simulink model "gridfor575V"  (R2015b)
settings: Solver=VariableStepAuto  StartTime=0.0  StopTime=10.0  RelTol=1e-3
values from neighbouring files (symbols this model uses):
  Ts = 5E-6    (= 5e-06)    [GE275103_inertial_support.m]
libraries: powerlib x8, sps_avr x1, powerlib_meascontrol x1
settings Model: Creator=Eren  LastModifiedBy=Eren

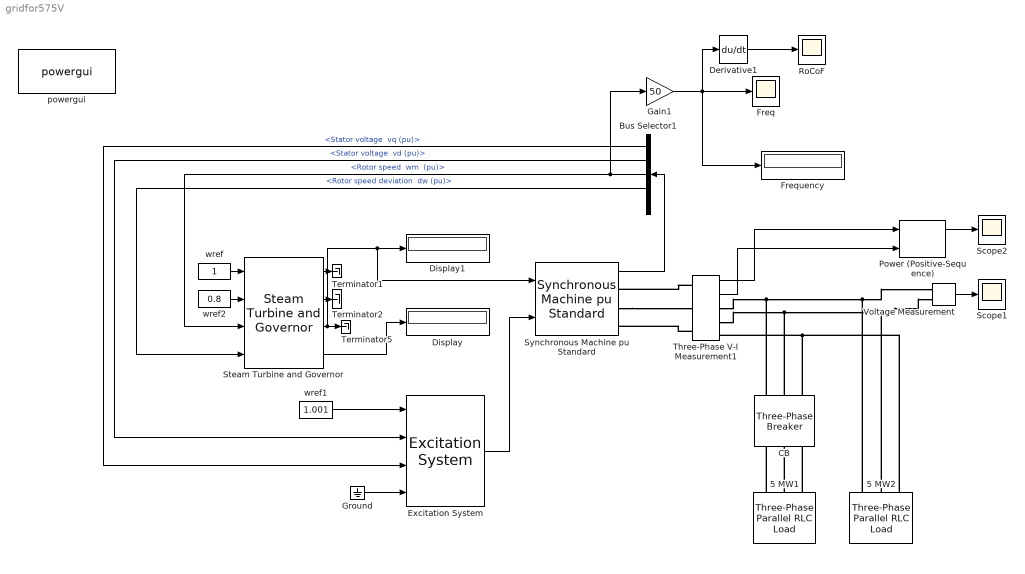
== system gridfor575V ==
  5 MW1 : powerlib/Elements/Three-Phase Parallel RLC Load  LConnTagsString=A|B|C  Configuration=Y (grounded)  NominalVoltage=575  Vabc=[1e3 1e3 1e3]  Vabcp=[1e3 1e3 1e3]  NominalFrequency=60  UnbalancedPower=off  ActivePower=5e5  InductivePower=0  CapacitivePower=0  Pabc=[10e3 9e3 11e3]  QLabc=[100 90 110]  QCabc=[100 90 110]  Pabcp=[10e3 9e3 11e3]  QLabcp=[100 90 110]  QCabcp=[100 90 110]  Measurements=None  LoadType=constant I
  5 MW2 : powerlib/Elements/Three-Phase Parallel RLC Load  LConnTagsString=A|B|C  Configuration=Y (grounded)  NominalVoltage=575  Vabc=[1e3 1e3 1e3]  Vabcp=[1e3 1e3 1e3]  NominalFrequency=60  UnbalancedPower=off  ActivePower=8e6  InductivePower=0  CapacitivePower=0  Pabc=[10e3 9e3 11e3]  QLabc=[100 90 110]  QCabc=[100 90 110]  Pabcp=[10e3 9e3 11e3]  QLabcp=[100 90 110]  QCabcp=[100 90 110]  Measurements=None  LoadType=constant PQ
  Bus Selector1 : BusSelector  OutputSignals="dq0 components.Stator voltage  vq (pu),dq0 components.Stator voltage  vd (pu),Mechanical.Rotor speed  wm  (pu),Mechanical.Rotor speed deviation  dw (pu),Output active power   Peo (pu)"
  CB : powerlib/Elements/Three-Phase Breaker  InitialState=open  SwitchA=on  SwitchB=on  SwitchC=on  SwitchTimes="[7  40]"  External=off  BreakerResistance=0.01  SnubberResistance=1e6  SnubberCapacitance=inf  Measurements=None
  Derivative1 : Derivative
  Display : Display
  Display1 : Display
  Excitation System : sps_avr/Excitation System  tr=20e-3  reg=[ 350, 0.001 ]  exc=[ 1, 0 ]  tgr=[ 0.1, 0.1 ]  damp=[ 0.001, 0.1 ]  sat=[ 0, 0 ]  lim=[ -11.5, 11.5, 0 ]  v0="[1.0  1.28]"
  Freq : Scope
  Frequency : Display
  Gain1 : Gain  Gain=50
  Ground : Ground
  Power (Positive-Sequence) : powerlib_meascontrol/Measurements/Power (Positive-Sequence)  Freq=50  Vinit=[0, 0]  Iinit=[0, 0]  Ts=0
  RoCoF : Scope
  Scope1 : Scope
  Scope2 : Scope
  Steam Turbine and Governor : powerlib/Machines/Steam Turbine and Governor  gentype=Tandem-compound (multi-mass)  reg1="[ 1.2  0.04    0 ]"  reg2="[ 0.001  0.15 ]"  reg3="[ -0.1  0.1  0  4.496]"  N=1800  turb1="[ 0  10   3.3   0.5   ]"  turb2="[ 0.5   0.5   0  0 ]"  HA="[  1.5498   0.24894  0  0 ]"  KA="[  83.47  42.702  0  0 ]"  DA="[  0.3104  0.05  0  0 ]*8"  ini1=250.35/555  ini2=[0.8,-120.13]
  Synchronous Machine pu Standard : powerlib/Machines/Synchronous Machine pu Standard  PresetModel=No  MechanicalLoad=Mechanical power Pm  ShowDetailedParameters=on  RotorType=Round  Units=per unit standard parameters  MeasurementBus=off  NominalParameters=[10e+06 575 60]  Reactances1=[ 1.81, 0.3, 0.23, 1.76, 0.65, 0.25, 0.15 ]  Reactances2=[2.24 0.17 0.12 1.02 0.13 0.08]  dAxisTimeConstants=Short-circuit  qAxisTimeConstants=Short-circuit  TimeConstants1="[ 4.4849  0.0681  0.1  ]"  TimeConstants2=[ 8.0, 0.03, 1.0, 0.07 ]  TimeConstants3="[  4.49  0.0681  0.0513  ]"  TimeConstants4=[ 8.0, 0.03, 0.3371, 0.0295 ]  TimeConstants5=[ 1.01, 0.053, 0.1 ]  TimeConstants6=[ 1.3201, 0.023, 1.0, 0.07 ]  TimeConstants7=[0.012 0.003 0.003]  TimeConstants8=[ 1.3201, 0.0231, 0.3371, 0.0295 ]  StatorResistance=0.037875  Mechanical=[5 0.02056 4]  PolePairs=20  InitialConditions="[ 0  0  0  0  0  0  0  0  1 ]"  SetSaturation=off  Saturation=[0.6404,0.7127,0.8441,0.9214,0.9956,1.082,1.19,1.316,1.457;0.7,0.7698,0.8872,0.9466,0.9969,1.046,1.1,1.151,1.201]  LoadFlowParameters=[1,0,0,0,0]  TsPowergui=0  TsBlock=-1  IterativeModel=Trapezoidal non iterative  BusType=swing  Pref=0  Qref=0  Qmin=-inf  Qmax=inf  PLF=0  QLF=0
  Terminator1 : Terminator
  Terminator2 : Terminator
  Terminator5 : Terminator
  Three-Phase V-I Measurement1 : powerlib/Measurements/Three-Phase V-I Measurement  VoltageMeasurement=phase-to-ground  SetLabelV=off  LabelV=Vsabc  Vpu=off  VpuLL=off  CurrentMeasurement=yes  SetLabelI=off  LabelI=Isabc  Ipu=off  Pbase=100e6  Vbase=690  OutputType=Complex  PhasorSimulation=off  PSBequivalent=0
  Voltage Measurement : powerlib/Measurements/Voltage Measurement  PhasorSimulation=off  OutputType=Complex  PSBequivalent=0
  powergui : powerlib/powergui  SimulationMode=Discrete  SolverType=Tustin/Backward Euler (TBE)  SampleTime=Ts  frequency=50  SPID=off  DisableSnubberDevices=off  DisableRonSwitches=off  DisableVfSwitches=off  SwTol=0  DisplayEquations=off  Interpol=off  ExternalGateDelay=off  methode=off  Ts=0  FunctionMessages=off  echomessages=off  HookPort=off  EnableUseOfTLC=off  x0status=blocks  frequencyindice=0  Pbase=100e6  ErrMax=1e-4  Iterations=50  UnitsV=kV  UnitsW=MW  buscounter=0  RestoreLinks=warning  ResistiveCurrentMeasurement=off  Frange=[0:2:500]  Ylog=off  Xlog=on  ShowGrid=off  save=off  variable=ZData  structure=0  ZoomFFT=on  StartTime=0.0  cycles=1  DisplayStyle=1  fundamental=60  FreqAxis=off  MaxFrequency=1000  frequencyindicesteady=1  RmsSteady=1  display=off
  wref : Constant
  wref1 : Constant  Value=1.001
  wref2 : Constant  Value=0.8
  wires:
  Synchronous Machine pu Standard/1 -> Bus Selector1/1
  Bus Selector1/3 -> Steam Turbine and Governor/3, Gain1/1  "<Rotor speed  wm  (pu)>"
  Bus Selector1/4 -> Steam Turbine and Governor/4  "<Rotor speed deviation  dw (pu)>"
  Excitation System/1 -> Synchronous Machine pu Standard/2
  Bus Selector1/2 -> Excitation System/2  "<Stator voltage  vd (pu)>"
  Bus Selector1/1 -> Excitation System/3  "<Stator voltage  vq (pu)>"
  Steam Turbine and Governor/3 -> Synchronous Machine pu Standard/1, Display1/1, Terminator5/1
  wref/1 -> Steam Turbine and Governor/1
  Ground/1 -> Excitation System/4
  wref1/1 -> Excitation System/1
  wref2/1 -> Steam Turbine and Governor/2
  Voltage Measurement/1 -> Scope1/1
  Three-Phase V-I Measurement1/1 -> Power (Positive-Sequence)/1
  Three-Phase V-I Measurement1/2 -> Power (Positive-Sequence)/2
  Power (Positive-Sequence)/1 -> Scope2/1
  Steam Turbine and Governor/1 -> Terminator1/1
  Steam Turbine and Governor/2 -> Terminator2/1
  Gain1/1 -> Derivative1/1, Frequency/1, Freq/1
  Derivative1/1 -> RoCoF/1
  Steam Turbine and Governor/4 -> Display/1
  connections:
  Three-Phase V-I Measurement1/RConn1 -- 5 MW2/LConn1 -- Voltage Measurement/LConn1 -- CB/RConn1
  Three-Phase V-I Measurement1/RConn2 -- 5 MW2/LConn2 -- Voltage Measurement/LConn2 -- CB/RConn2
  5 MW2/LConn3 -- CB/RConn3 -- Three-Phase V-I Measurement1/RConn3
  5 MW1/LConn3 -- CB/LConn3
  Three-Phase V-I Measurement1/LConn1 -- Synchronous Machine pu Standard/RConn1
  5 MW1/LConn2 -- CB/LConn2
  Three-Phase V-I Measurement1/LConn3 -- Synchronous Machine pu Standard/RConn3
  5 MW1/LConn1 -- CB/LConn1
  Synchronous Machine pu Standard/RConn2 -- Three-Phase V-I Measurement1/LConn2
